simulink model "MEE6044_FKM_DWMR_20MAI0001_jcomp1"  (R2020b)
settings: Solver=VariableStepAuto  StartTime=0.0  StopTime=210.2656  RelTol=1e-3
undefined symbols (not defined in the file): sigbuilder_block
libraries: simulink_extras x1, simulink x1
settings Model: Creator=rikav  LastModifiedBy=rikav

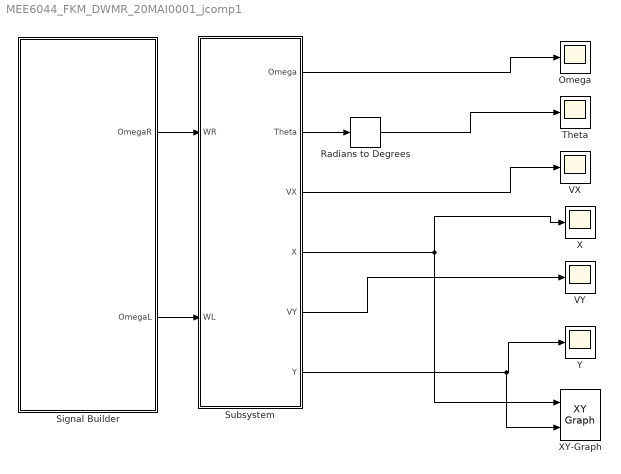
== system MEE6044_FKM_DWMR_20MAI0001_jcomp1 ==
  Omega : Scope
  Radians to Degrees : simulink_extras/Transformations/Radians to Degrees
  Signal Builder : Subsystem  Tag=STV Subsys  LoadFcn=sigbuilder_block('load');  StartFcn=sigbuilder_block('start');  StopFcn=sigbuilder_block('stop');  ClipboardFcn=sigbuilder_block('clipboard');  mask(Sigbuilder block){tuvar=[0:10]}
      mask help: Simulink:masks:SigbuilderBlock_MD
      mask init:
      | if ~strcmp(get_param(bdroot(gcbh),'SimulationStatus'),'stopped') tuvar = sigbuilder_block('maskInit'); end
      settings: CopyFcn=sigbuilder_block('copy');  DeleteFcn=sigbuilder_block('delete');  ModelCloseFcn=sigbuilder_block('modelClose');  PreSaveFcn=sigbuilder_block('preSave');  PauseFcn=sigbuilder_block('pause');  ContinueFcn=sigbuilder_block('continue');  NameChangeFcn=sigbuilder_block('namechange');  OpenFcn=sigbuilder_block('open',[5.4 141.6 1141.2 444.6 ]);  CloseFcn=sigbuilder_block('close');
      mask Display: plot(0, 0, 100, 100,[2, 2, 32, 32, 2], [68, 8, 8, 68, 68],[32, 2], [38, 38], [32, 19, 2],[53, 60, 44], [32, 17, 17, 2],[16, 16, 31, 31]);txt = getActiveGroup(gcbh);text(2, 100, txt,'verticalAlignment', 'top');
  Subsystem : Subsystem
  Theta : Scope
  VX : Scope
  VY : Scope
  X : Scope
  XY-Graph : simulink/Sinks/XY Graph  xmin=-100  xmax=1500  ymin=-100  ymax=1500  st=-1
  Y : Scope
  wires:
  Subsystem/1(Omega) -> Omega/1
  Subsystem/3(VX) -> VX/1
  Subsystem/4(X) -> XY-Graph/1, X/1
  Subsystem/5(VY) -> VY/1
  Subsystem/6(Y) -> XY-Graph/2, Y/1
  Subsystem/2(Theta) -> Radians to Degrees/1
  Radians to Degrees/1 -> Theta/1
  Signal Builder/2(OmegaL) -> Subsystem/2(WL)
  Signal Builder/1(OmegaR) -> Subsystem/1(WR)

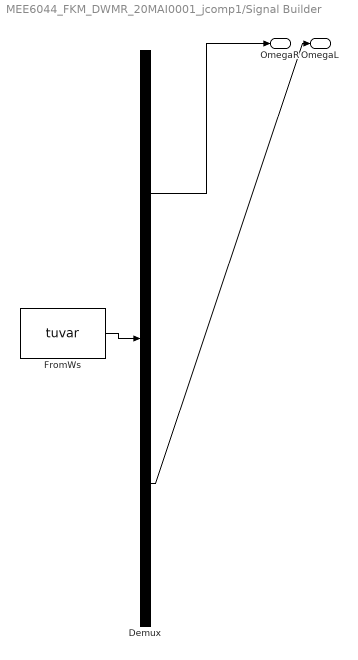
== system MEE6044_FKM_DWMR_20MAI0001_jcomp1/Signal Builder ==
  Demux : Demux  Tag=STV Demux  Outputs=2
      settings: DisplayOption=none
  FromWs : FromWorkspace  Tag=STV FromWs  VariableName=tuvar
      SigBuilderData=|
      | common.afterFinalStr = 'Extrapolate'
      | common.sampleTime = 0
      | dataSet.timeRange = [0 52.5664]
      | dataSet.name = 'Group 1'
      | sbobj.Groups.Name = 'Group 1'
      | sbobj.Groups.Signals(1).Name = 'OmegaR'
      | sbobj.Groups.Signals(1).XData = [0 10 10 13.1416 13.1416 23.1416 23.1416 26.2832 26.2832 36.2832 36.2832 39.4248 39.4248 49.4248 49.4248 52.5664]
      | sbobj.Groups.Signals(1).YData = [1 1 0.5 0.5 1 1 0.5 0.5 1 1 0.5 0.5 1 1 0.5 0.5]
      | sbobj.Groups.Signals(2).Name = 'OmegaL'
      | sbobj.Groups.Signals(2).XData = [0 10 10 13.1416 13.1416 23.1416 23.1416 26.2832 26.2832 36.2832 36.2832 39.4248 39.4248 49.4248 49.4248 52.5664]
      | sbobj.Groups.Signals(2).YData = [1 1 -0.5 -0.5 1 1 -0.5 -0.5 1 1 -0.5 -0.5 1 1 -0.5 -0.5]
      | sbobj.Groups.TimeRange = [0 52.5664]
  OmegaR : Outport  Tag=STV Outport
  OmegaL : Outport  Tag=STV Outport  Port=2
  wires:
  FromWs/1 -> Demux/1
  Demux/1 -> OmegaR/1
  Demux/2 -> OmegaL/1

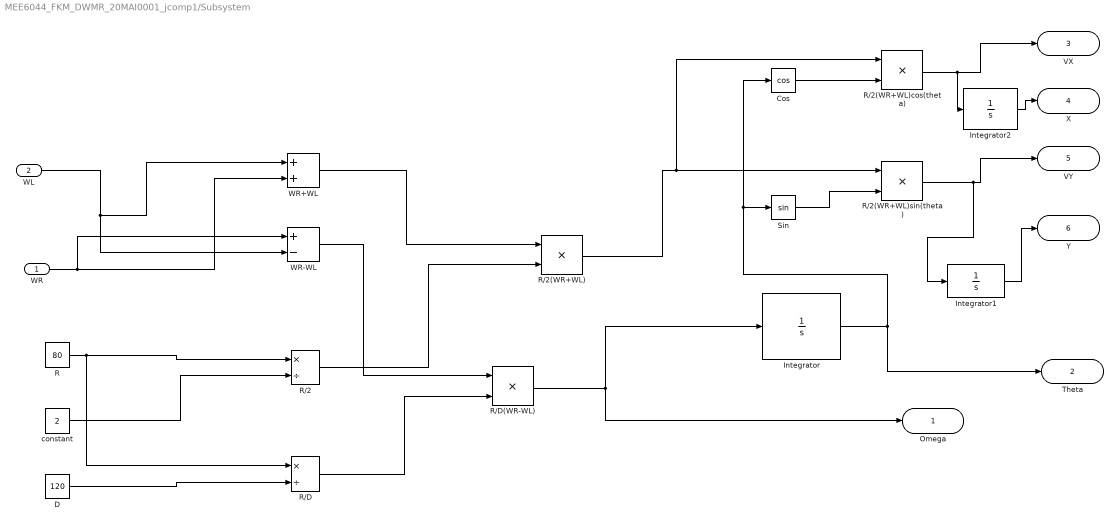
== system MEE6044_FKM_DWMR_20MAI0001_jcomp1/Subsystem ==
  WR : Inport
  WL : Inport  Port=2
  Cos : Trigonometry  Operator=cos
  D : Constant  Value=120
  Integrator : Integrator
  Integrator1 : Integrator
  Integrator2 : Integrator
  R : Constant  Value=80
  R/2 : Product  Inputs=*/
  R/2(WR+WL) : Product
  R/2(WR+WL)cos(theta) : Product
  R/2(WR+WL)sin(theta) : Product
  R/D : Product  Inputs=*/
  R/D(WR-WL) : Product
  Sin : Trigonometry
  WR+WL : Sum
  WR-WL : Sum  Inputs=+-
  constant : Constant  Value=2
  Omega : Outport
  Theta : Outport  Port=2
  VX : Outport  Port=3
  X : Outport  Port=4
  VY : Outport  Port=5
  Y : Outport  Port=6
  wires:
  WL/1 -> WR-WL/2, WR+WL/1
  WR/1 -> WR-WL/1, WR+WL/2
  R/1 -> R/D/1, R/2/1
  constant/1 -> R/2/2
  D/1 -> R/D/2
  WR+WL/1 -> R/2(WR+WL)/1
  R/2/1 -> R/2(WR+WL)/2
  WR-WL/1 -> R/D(WR-WL)/1
  R/D/1 -> R/D(WR-WL)/2
  R/D(WR-WL)/1 -> Omega/1, Integrator/1
  Integrator/1 -> Cos/1, Sin/1, Theta/1
  Cos/1 -> R/2(WR+WL)cos(theta)/2
  Sin/1 -> R/2(WR+WL)sin(theta)/2
  R/2(WR+WL)/1 -> R/2(WR+WL)cos(theta)/1, R/2(WR+WL)sin(theta)/1
  R/2(WR+WL)cos(theta)/1 -> Integrator2/1, VX/1
  R/2(WR+WL)sin(theta)/1 -> Integrator1/1, VY/1
  Integrator2/1 -> X/1
  Integrator1/1 -> Y/1
